simulink model "bh_CONTROL_4dof_manip_swing_balance"  (R2017a)
settings: Solver=ode4  StartTime=0.0  StopTime=44  FixedStep=0.001  RelTol=1e-5
values from neighbouring files (symbols this model uses):
  b3_damp = res_T.b3_damp    [bh_pend_solve_ODE_sys.m]
  g = res_T.g    [bh_pend_solve_ODE_sys.m]    (also in bh_pend_solve_ODE_sys_custom.m)
  Io3_xx = res_T.Io3_xx    [bh_pend_solve_ODE_sys.m]
  L3y = res_T.L3y    [bh_pend_solve_ODE_sys.m]    (also in bh_pend_solve_ODE_sys_custom.m)
  m = res_T.mass3    [bh_pend_solve_ODE_sys_custom.m]
  mass3 = res_T.mass3    [bh_pend_solve_ODE_sys.m]    (also in bh_pend_solve_ODE_sys_custom.m)
  N = 1 + N_steps    [bh_pend_solve_ODE_sys_custom.m]
undefined symbols (not defined in the file or in its folder): b1_damp, b2_damp, b4_damp, Hz, L1x, L1y, L1z, L2x, L2y, L2z, L3x, L3z, mass1, mass2, mass4, Rturn, theta1_0, theta1_dot_0, theta2_0, theta2_dot_0, theta3_0, theta3_dot_0, theta4_0, theta4_dot_0, X, Y, Z
libraries: simulink_extras x43, sm_lib x26, nesl_utility x24, simulink x7
(part 3 of 3)

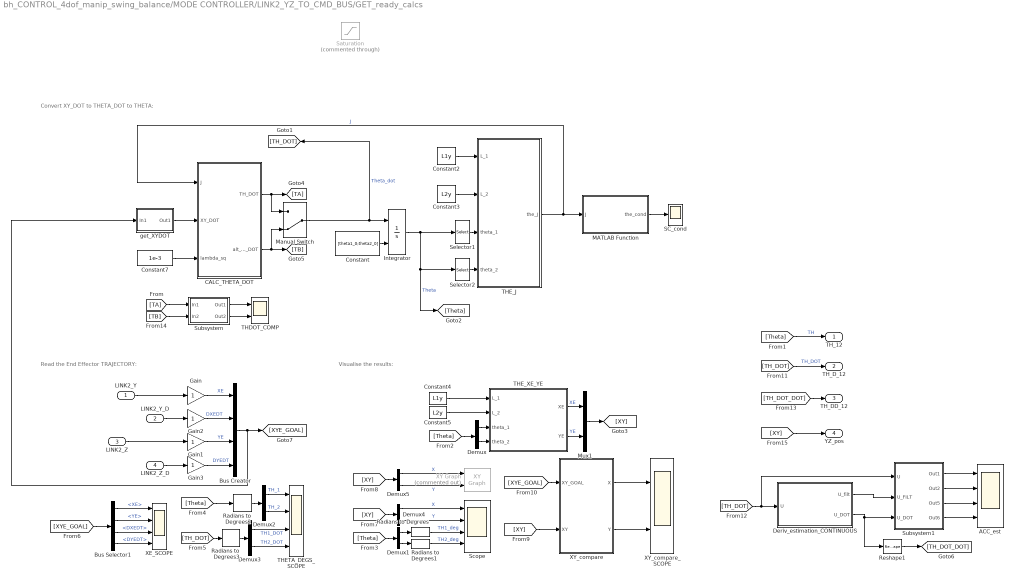
== system bh_CONTROL_4dof_manip_swing_balance/MODE CONTROLLER/LINK2_YZ_TO_CMD_BUS/GET_ready_calcs ==
  note: Visualise the results:
  note: Convert XY_DOT to THETA_DOT to THETA:
  note: Read the End Effector TRAJECTORY:
  LINK2_Y : Inport
  LINK2_Y_D : Inport  Port=2
  LINK2_Z : Inport  Port=3
  LINK2_Z_D : Inport  Port=4
  ACC_est : Scope  NumInputPorts=4
  Bus Creator : BusCreator  Inputs=4
  Bus Selector1 : BusSelector  OutputSignals=XE,YE,DXEDT,DYEDT
  CALC_THETA_DOT : MATLAB Function  TreatAsAtomicUnit=on
  Constant : Constant  Value=[theta1_0;theta2_0]  VectorParams1D=off
  Constant2 : Constant  Value=L1y
  Constant3 : Constant  Value=L2y
  Constant4 : Constant  Value=L1y
  Constant5 : Constant  Value=L2y
  Constant7 : Constant  Value=1e-3
  Demux{,1..5} (6 alike) : Demux  Outputs=2
  Deriv_estimation_CONTINUOUS : Subsystem  mask(Derivative Estimation){wn=2*pi*100, p=1, x0_val=0, v0_val=0}
      mask prompts: wn "Natural frequency, wn (rad/sec)"; p "Damping ratio, p"; x0_val "X_IC"; v0_val "X_DOT_IC"
      mask help:
      | A simple derivative estimator using a 2nd order representation between input and output.
      |
      | The integrators use a discrete FORWARd Euler rule, and a sample time needs to be specified.
      mask init:
      | str0 = sprintf('fn = %.2f [Hz]', (wn/(2*pi)));
      | str1 = sprintf('wn = %.2f', wn);
      | str2 = sprintf('p  = %.3g', p);
      | %str3 = sprintf('dt = %.2g', dt);
      | str = char(str0,str1,str2);
      mask Display: disp(str)
  Gain{,1..3} (4 alike) : Gain
  Integrator : Integrator  InitialConditionSource=external
  MATLAB Function : MATLAB Function  TreatAsAtomicUnit=on
  Manual Switch : ManualSwitch  CurrentSetting=0
  Mux1 : Mux  Inputs=2
  Radians to Degrees{,1..3} (4 alike) : simulink_extras/Transformations/Radians to Degrees
  Reshape1 : Reshape  OutputDimensionality=Column vector (2-D)
  SC_cond : Scope
  Saturation : Saturate  Commented=through  UpperLimit=6  LowerLimit=-6
  Scope : Scope  NumInputPorts=4
  Selector1 : Selector  InputPortWidth=2  IndexOptions=Index vector (dialog)  Indices=1  OutputSizes=1
  Selector2 : Selector  InputPortWidth=2  IndexOptions=Index vector (dialog)  Indices=2  OutputSizes=1
  Subsystem : Subsystem
  Subsystem1 : Subsystem
  THDOT_COMP : Scope  NumInputPorts=2
  THETA_DEGS_SCOPE : Scope  NumInputPorts=4
  THE_J : MATLAB Function  TreatAsAtomicUnit=on
  THE_XE_YE : MATLAB Function  TreatAsAtomicUnit=on
  XE_SCOPE : Scope  NumInputPorts=4
  XY Graph : simulink/Sinks/XY Graph  Commented=on  xmin=0  xmax=1.6  ymin=0  ymax=1.6  st=-1
  XY_compare : Subsystem
  XY_compare_SCOPE : Scope  NumInputPorts=2
  get_XYDOT : Subsystem
  TH_12 : Outport
  TH_D_12 : Outport  Port=2
  TH_DD_12 : Outport  Port=3
  YZ_pos : Outport  Port=4
  wires:
  XY_compare/1(X) -> XY_compare_SCOPE/1
  Constant7/1 -> CALC_THETA_DOT/3(lambda_sq)
  [XY] -> XY_compare/2(XY)
  Constant3/1 -> THE_J/2(L_2)
  Bus Selector1/2 -> XE_SCOPE/2  "<YE>"
  Subsystem/2(Out2) -> THDOT_COMP/2
  [Theta] -> Radians to Degrees2/1
  Mux1/1 -> [XY]
  Subsystem/1(Out1) -> THDOT_COMP/1
  Demux3/2 -> THETA_DEGS_SCOPE/4  "TH2_DOT"
  CALC_THETA_DOT/1(TH_DOT) -> [TA], Manual Switch/1
  [Theta] -> Demux/1
  [TB] -> Subsystem/2(In2)
  [TA] -> Subsystem/1(In1)
  Radians to Degrees1/1 -> Scope/4  "TH2_deg"
  Constant2/1 -> THE_J/1(L_1)
  CALC_THETA_DOT/2(alt_TH_DOT) -> [TB], Manual Switch/2
  XY_compare/2(Y) -> XY_compare_SCOPE/2
  THE_J/1(the_J) -> CALC_THETA_DOT/1(J), MATLAB Function/1(J)  "J"
  Radians to Degrees2/1 -> Demux2/1
  Demux5/2 -> XY Graph/2  "Y"
  [XYE_GOAL] -> XY_compare/1(XY_GOAL)
  Constant/1 -> Integrator/2
  Bus Creator/1 -> get_XYDOT/1(In1), [XYE_GOAL]
  Radians to Degrees3/1 -> Demux3/1
  Constant5/1 -> THE_XE_YE/2(L_2)
  Bus Selector1/3 -> XE_SCOPE/3  "<DXEDT>"
  Bus Selector1/4 -> XE_SCOPE/4  "<DYEDT>"
  Demux4/2 -> Scope/2  "Y"
  Demux1/1 -> Radians to Degrees/1
  Radians to Degrees/1 -> Scope/3  "TH1_deg"
  get_XYDOT/1(Out1) -> CALC_THETA_DOT/2(XY_DOT)
  Bus Selector1/1 -> XE_SCOPE/1  "<XE>"
  [XYE_GOAL] -> Bus Selector1/1
  Demux3/1 -> THETA_DEGS_SCOPE/3  "TH1_DOT"
  [TH_DOT] -> Radians to Degrees3/1
  Demux2/2 -> THETA_DEGS_SCOPE/2  "TH_2"
  [Theta] -> Demux1/1
  [XY] -> Demux5/1
  MATLAB Function/1(the_cond) -> SC_cond/1
  Demux/1 -> THE_XE_YE/3(theta_1)
  THE_XE_YE/2(YE) -> Mux1/2  "YE"
  Selector1/1 -> THE_J/3(theta_1)
  Selector2/1 -> THE_J/4(theta_2)
  Demux2/1 -> THETA_DEGS_SCOPE/1  "TH_1"
  Demux5/1 -> XY Graph/1  "X"
  Integrator/1 -> Selector2/1, [Theta], Selector1/1  "Theta"
  THE_XE_YE/1(XE) -> Mux1/1  "XE"
  [XY] -> Demux4/1
  Constant4/1 -> THE_XE_YE/1(L_1)
  Demux4/1 -> Scope/1  "X"
  Manual Switch/1 -> [TH_DOT], Integrator/1  "Theta_dot"
  Demux/2 -> THE_XE_YE/4(theta_2)
  Demux1/2 -> Radians to Degrees1/1
  [TH_DOT] -> TH_D_12/1  "TH_DOT"
  [Theta] -> TH_12/1  "TH"
  Deriv_estimation_CONTINUOUS/2(U_DOT) -> Reshape1/1, Subsystem1/3(U_DOT)
  Deriv_estimation_CONTINUOUS/1(U_filt) -> Subsystem1/2(U_FILT)
  [TH_DOT] -> Subsystem1/1(U), Deriv_estimation_CONTINUOUS/1(U)
  Reshape1/1 -> [TH_DOT_DOT]
  Subsystem1/1(Out1) -> ACC_est/1
  Subsystem1/2(Out2) -> ACC_est/2
  Subsystem1/3(Out5) -> ACC_est/3
  Subsystem1/4(Out6) -> ACC_est/4
  [TH_DOT_DOT] -> TH_DD_12/1
  Gain1/1 -> Bus Creator/3  "YE"
  Gain2/1 -> Bus Creator/2  "DXEDT"
  Gain3/1 -> Bus Creator/4  "DYEDT"
  Gain/1 -> Bus Creator/1  "XE"
  LINK2_Y/1 -> Gain/1
  LINK2_Z/1 -> Gain1/1
  LINK2_Z_D/1 -> Gain3/1
  LINK2_Y_D/1 -> Gain2/1
  [XY] -> YZ_pos/1

== system bh_CONTROL_4dof_manip_swing_balance/MODE CONTROLLER/STATE_CONTROL/BIRTH_calcs ==
  Enable : EnablePort
  Bus Creator : BusCreator  Inputs=4  OutDataTypeStr=Bus: BUS_DEF_2LINK_TRAJ
  Constant2 : Constant  Value=L1y + L2y
  Constant3 : Constant  Value=0
  Constant4 : Constant  Value=0
  Constant5 : Constant  Value=0
  LINK2_EFF_TRAJ : Outport  OutDataTypeStr=Bus: BUS_DEF_2LINK_TRAJ
  wires:
  Constant5/1 -> Bus Creator/3  "LINK2_EFF_Z_D"
  Constant2/1 -> Bus Creator/2  "LINK2_EFF_Y"
  Constant3/1 -> Bus Creator/4  "LINK2_EFF_Z"
  Constant4/1 -> Bus Creator/1  "LINK2_EFF_Y_D"
  Bus Creator/1 -> LINK2_EFF_TRAJ/1

== system bh_CONTROL_4dof_manip_swing_balance/MODE CONTROLLER/STATE_CONTROL/DO_BALANCE_calcs ==
  PMB : Inport
  Y2B : Inport  Port=2
  y_at start : Inport  Port=3
  yD_at start : Inport  Port=4
  Enable : EnablePort
  Bus Creator : BusCreator  Inputs=4  OutDataTypeStr=Bus: BUS_DEF_2LINK_TRAJ
  Constant3 : Constant  Value=0
  Constant5 : Constant  Value=0
  DO_BALANCE_sys : Subsystem  TreatAsAtomicUnit=on
  Gain1 : Gain
  Gain2 : Gain
  Scope1 : Scope
  Terminator : Terminator
  LINK2_EFF_TRAJ : Outport  OutDataTypeStr=Bus: BUS_DEF_2LINK_TRAJ
  wires:
  PMB/1 -> DO_BALANCE_sys/1(PMB)
  Y2B/1 -> DO_BALANCE_sys/2(Y2B)
  Gain1/1 -> Bus Creator/1  "LINK2_EFF_Y_D"
  Bus Creator/1 -> LINK2_EFF_TRAJ/1
  Gain2/1 -> Scope1/1, Bus Creator/2  "LINK2_EFF_Y"
  Constant5/1 -> Bus Creator/3  "LINK2_EFF_Z_D"
  Constant3/1 -> Bus Creator/4  "LINK2_EFF_Z"
  DO_BALANCE_sys/2(P) -> Gain2/1
  DO_BALANCE_sys/1(V) -> Gain1/1
  y_at start/1 -> DO_BALANCE_sys/3(y_at start)
  DO_BALANCE_sys/3(A) -> Terminator/1
  yD_at start/1 -> DO_BALANCE_sys/4(yD_at start)

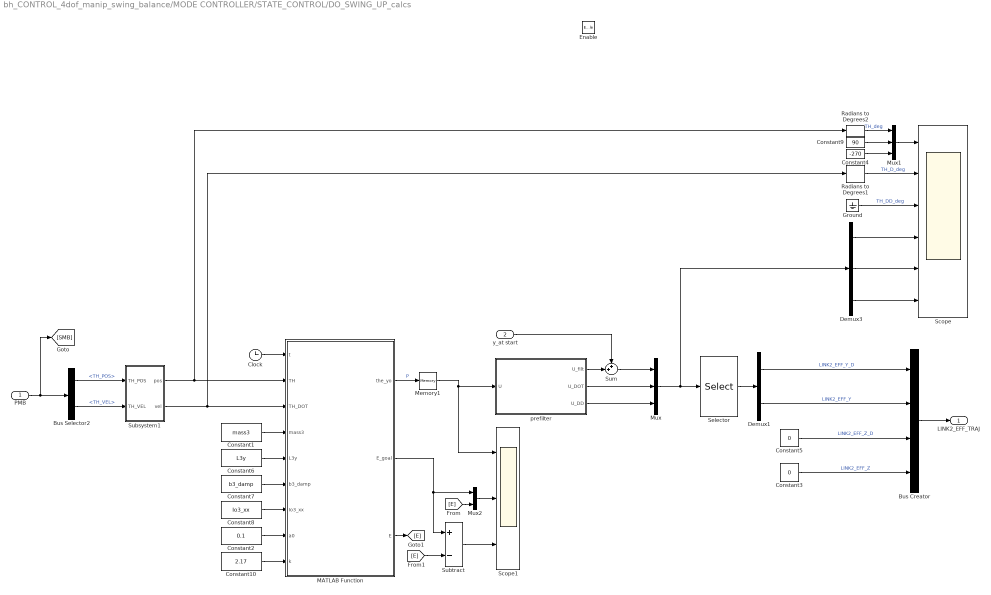
== system bh_CONTROL_4dof_manip_swing_balance/MODE CONTROLLER/STATE_CONTROL/DO_SWING_UP_calcs ==
  PMB : Inport
  y_at start : Inport  Port=2
  Enable : EnablePort
  Bus Creator : BusCreator  Inputs=4  OutDataTypeStr=Bus: BUS_DEF_2LINK_TRAJ
  Bus Selector2 : BusSelector  OutputSignals=MEAS_BUS.TH_POS,MEAS_BUS.TH_VEL
  Clock : Clock
  Constant1 : Constant  Value=mass3
  Constant10 : Constant  Value=2.17
  Constant2 : Constant  Value=0.1
  Constant3 : Constant  Value=0
  Constant4 : Constant  Value=-270
  Constant5 : Constant  Value=0
  Constant6 : Constant  Value=L3y
  Constant7 : Constant  Value=b3_damp
  Constant8 : Constant  Value=Io3_xx
  Constant9 : Constant  Value=90
  Demux1 : Demux  Outputs=2
  Demux3 : Demux  Outputs=3
  Ground : Ground
  MATLAB Function : MATLAB Function  TreatAsAtomicUnit=on
  Memory1 : Memory
  Mux : Mux  Inputs=3
  Mux1 : Mux  Inputs=3
  Mux2 : Mux  Inputs=2
  Radians to Degrees1 : simulink_extras/Transformations/Radians to Degrees
  Radians to Degrees2 : simulink_extras/Transformations/Radians to Degrees
  Scope : Scope  NumInputPorts=6
  Scope1 : Scope  NumInputPorts=3
  Selector : Selector  InputPortWidth=3  IndexOptions=Index vector (dialog)  Indices=[2 1]  OutputSizes=1
  Subsystem1 : Subsystem
  Subtract : Sum  Inputs=+-
  Sum : Sum  Inputs=++|
  prefilter : Subsystem  mask(Derivative Estimation){wn=2*pi*35, p=0.95}
      mask prompts: wn "Natural frequency, wn (rad/sec)"; p "Damping ratio, p"
      mask help:
      | A simple derivative estimator using a 2nd order representation between input and output.
      |
      | The integrators use a discrete FORWARd Euler rule, and a sample time needs to be specified.
      mask init:
      | str1 = sprintf('wn = %.2f', wn);
      | str2 = sprintf('p  = %.2f', p);
      | %str3 = sprintf('dt = %.2f', dt);
      | %str = char(str1,str2,str3);
      | %str3 = sprintf('dt = %.2f', dt);
      | str = char(str1,str2);
      mask Display: disp(str)
  LINK2_EFF_TRAJ : Outport  OutDataTypeStr=Bus: BUS_DEF_2LINK_TRAJ
  wires:
  Demux1/2 -> Bus Creator/2  "LINK2_EFF_Y"
  Demux1/1 -> Bus Creator/1  "LINK2_EFF_Y_D"
  Constant5/1 -> Bus Creator/3  "LINK2_EFF_Z_D"
  Constant3/1 -> Bus Creator/4  "LINK2_EFF_Z"
  Bus Creator/1 -> LINK2_EFF_TRAJ/1
  Clock/1 -> MATLAB Function/1(t)
  Mux1/1 -> Scope/1
  Constant10/1 -> MATLAB Function/9(k)
  Mux2/1 -> Scope1/2
  Demux3/2 -> Scope/5
  Constant6/1 -> MATLAB Function/5(L3y)
  Subtract/1 -> Scope1/3
  prefilter/1(U_filt) -> Sum/2
  prefilter/3(U_DD) -> Mux/3
  Constant8/1 -> MATLAB Function/7(Io3_xx)
  Ground/1 -> Scope/3  "TH_DD_deg"
  MATLAB Function/2(E_goal) -> Mux2/1, Subtract/1
  Demux3/3 -> Scope/6
  Constant7/1 -> MATLAB Function/6(b3_damp)
  Constant1/1 -> MATLAB Function/4(mass3)
  Constant2/1 -> MATLAB Function/8(a0)
  Constant9/1 -> Mux1/2
  Demux3/1 -> Scope/4
  Radians to Degrees2/1 -> Mux1/1  "TH_deg"
  MATLAB Function/1(the_yo) -> Memory1/1  "P"
  Radians to Degrees1/1 -> Scope/2  "TH_D_deg"
  prefilter/2(U_DOT) -> Mux/2
  PMB/1 -> [SMB], Bus Selector2/1
  Mux/1 -> Selector/1, Demux3/1
  Bus Selector2/1 -> Subsystem1/1(TH_POS)  "<TH_POS>"
  Bus Selector2/2 -> Subsystem1/2(TH_VEL)  "<TH_VEL>"
  Subsystem1/1(pos) -> MATLAB Function/2(TH), Radians to Degrees2/1
  Subsystem1/2(vel) -> MATLAB Function/3(TH_DOT), Radians to Degrees1/1
  Sum/1 -> Mux/1
  y_at start/1 -> Sum/1
  Selector/1 -> Demux1/1
  Constant4/1 -> Mux1/3
  Memory1/1 -> prefilter/1(U), Scope1/1
  MATLAB Function/3(E) -> [E]
  [E] -> Subtract/2
  [E] -> Mux2/2

== system bh_CONTROL_4dof_manip_swing_balance/MODE CONTROLLER/STATE_CONTROL/DO_moving_to_ready_calcs ==
  Enable : EnablePort
  BIRTH_moves_to_READY1 : Subsystem
  LINK2_traj : Outport  OutDataTypeStr=Bus: BUS_DEF_2LINK_TRAJ
  wires:
  BIRTH_moves_to_READY1/1(LINK2_EFF_TRAJ) -> LINK2_traj/1

== system bh_CONTROL_4dof_manip_swing_balance/MODE CONTROLLER/STATE_CONTROL/Subsystem ==
  PMB : Inport
  Bus Creator : BusCreator  Inputs=2
  Bus Selector : BusSelector  OutputSignals=MEAS_BUS.TH_POS
  Demux : Demux  Outputs=2
  Deriv_estimation_CONTINUOUS : Subsystem  mask(Derivative Estimation){wn=2*pi*100, p=1, x0_val=0, v0_val=0}
      mask prompts: wn "Natural frequency, wn (rad/sec)"; p "Damping ratio, p"; x0_val "X_IC"; v0_val "X_DOT_IC"
      mask help:
      | A simple derivative estimator using a 2nd order representation between input and output.
      |
      | The integrators use a discrete FORWARd Euler rule, and a sample time needs to be specified.
      mask init:
      | str0 = sprintf('fn = %.2f [Hz]', (wn/(2*pi)));
      | str1 = sprintf('wn = %.2f', wn);
      | str2 = sprintf('p  = %.3g', p);
      | %str3 = sprintf('dt = %.2g', dt);
      | str = char(str0,str1,str2);
      mask Display: disp(str)
  LINK2_EFF_YZ_from_THETA : Subsystem
  Selector1 : Selector  InputPortWidth=4  IndexOptions=Index vector (dialog)  Indices=[1,2]  OutputSizes=1
  Terminator : Terminator
  Terminator1 : Terminator
  Y2 : Outport
  Y2_D : Outport  Port=2
  Y2_Bus : Outport  Port=3
  wires:
  PMB/1 -> Bus Selector/1
  Bus Selector/1 -> Selector1/1  "<TH_POS>"
  Selector1/1 -> Demux/1
  Demux/1 -> LINK2_EFF_YZ_from_THETA/1(TH1)
  Demux/2 -> LINK2_EFF_YZ_from_THETA/2(TH2)
  LINK2_EFF_YZ_from_THETA/2(Z2_EFF) -> Terminator/1
  LINK2_EFF_YZ_from_THETA/1(Y2_EFF) -> Deriv_estimation_CONTINUOUS/1(U), Bus Creator/1, Y2/1  "Y2"
  Deriv_estimation_CONTINUOUS/1(U_filt) -> Terminator1/1
  Bus Creator/1 -> Y2_Bus/1
  Deriv_estimation_CONTINUOUS/2(U_DOT) -> Y2_D/1, Bus Creator/2  "Y2_D"

== system bh_CONTROL_4dof_manip_swing_balance/MODE CONTROLLER/STATE_CONTROL/Subsystem1 ==
  TH_POS : Inport
  TH_VEL : Inport  Port=2
  Mux : Mux  Inputs=2
  Selector1 : Selector  InputPortWidth=4  IndexOptions=Index vector (dialog)  Indices=[1 2 3]  OutputSizes=1
  Selector2 : Selector  InputPortWidth=4  IndexOptions=Index vector (dialog)  Indices=[1 2 3]  OutputSizes=1
  Sum of Elements : Sum  Inputs=+
  Sum of Elements1 : Sum  Inputs=+
  pos : Outport
  vel : Outport  Port=2
  PV : Outport  Port=3
  wires:
  TH_POS/1 -> Selector2/1
  Sum of Elements/1 -> Mux/1, pos/1
  Selector2/1 -> Sum of Elements/1
  TH_VEL/1 -> Selector1/1
  Selector1/1 -> Sum of Elements1/1
  Sum of Elements1/1 -> Mux/2, vel/1
  Mux/1 -> PV/1

== system bh_CONTROL_4dof_manip_swing_balance/SIMULINK_MODEL/inside_MCKGQ/Subsystem ==
  iTH1 : Inport
  iTH2 : Inport  Port=2
  iTH3 : Inport  Port=3
  iTH4 : Inport  Port=4
  iTH1D : Inport  Port=5
  iTH2D : Inport  Port=6
  iTH3D : Inport  Port=7
  iTH4D : Inport  Port=8
  Bus Creator : BusCreator  Inputs=10
  Bus Selector : BusSelector  OutputSignals=TH1,TH2,TH3,TH4,TH1D,TH2D,TH3D,TH4D
  Mux : Mux
  Mux1 : Mux
  Reshape : Reshape  OutputDimensionality=Column vector (2-D)
  Reshape1 : Reshape  OutputDimensionality=Column vector (2-D)
  Terminator : Terminator
  TH1 : Outport
  TH2 : Outport  Port=2
  TH3 : Outport  Port=3
  TH1D : Outport  Port=4
  TH2D : Outport  Port=5
  TH3D : Outport  Port=6
  TH4D : Outport  Port=7
  TH_BUS : Outport  Port=8
  wires:
  iTH2/1 -> Bus Creator/3, Mux/2  "TH2"
  iTH1/1 -> Bus Creator/2, Mux/1  "TH1"
  iTH2D/1 -> Bus Creator/7, Mux1/2  "TH2D"
  iTH1D/1 -> Bus Creator/6, Mux1/1  "TH1D"
  Mux/1 -> Reshape/1
  Mux1/1 -> Reshape1/1
  Reshape/1 -> Bus Creator/1  "theta_col"
  Reshape1/1 -> Bus Creator/10  "theta_DOT_col"
  Bus Creator/1 -> TH_BUS/1, Bus Selector/1
  iTH3D/1 -> Bus Creator/8, Mux1/3  "TH3D"
  iTH3/1 -> Bus Creator/4, Mux/3  "TH3"
  Bus Selector/1 -> TH1/1  "<TH1>"
  Bus Selector/2 -> TH2/1  "<TH2>"
  Bus Selector/3 -> TH3/1  "<TH3>"
  Bus Selector/5 -> TH1D/1  "<TH1D>"
  Bus Selector/6 -> TH2D/1  "<TH2D>"
  Bus Selector/7 -> TH3D/1  "<TH3D>"
  iTH4/1 -> Bus Creator/5, Mux/4  "TH4"
  iTH4D/1 -> Bus Creator/9, Mux1/4  "TH4D"
  Bus Selector/4 -> Terminator/1  "<TH4>"
  Bus Selector/8 -> TH4D/1  "<TH4D>"

== system bh_CONTROL_4dof_manip_swing_balance/SIMULINK_MODEL/inside_MCKGQ/Subsystem1 ==
  M : Inport
  C : Inport  Port=2
  K : Inport  Port=3
  G : Inport  Port=4
  Q : Inport  Port=5
  T : Inport  Port=6
  Bus Selector : BusSelector  OutputSignals=theta_DOT_col
  Bus Selector1 : BusSelector  OutputSignals=theta_col
  Demux : Demux
  MATLAB Function : MATLAB Function  TreatAsAtomicUnit=on
  Product : Product  Multiplication=Matrix(*)
  Product1 : Product  Multiplication=Matrix(*)
  Product2 : Product  Inputs=/  Multiplication=Matrix(*)
  Product3 : Product  Multiplication=Matrix(*)
  SC_cond : Scope
  Sum : Sum  Inputs=+|+|+
  Sum1 : Sum  Inputs=|-+
  TH1_DD : Outport
  TH2_DD : Outport  Port=2
  TH3_DD : Outport  Port=3
  TH4_DD : Outport  Port=4
  wires:
  T/1 -> [T]
  C/1 -> Product/1
  [T] -> Bus Selector/1
  Bus Selector/1 -> Product/2  "<theta_DOT_col>"
  K/1 -> Product1/1
  [T] -> Bus Selector1/1
  Bus Selector1/1 -> Product1/2  "<theta_col>"
  Q/1 -> Sum1/2
  Product1/1 -> Sum/2
  G/1 -> Sum/3
  Product/1 -> Sum/1
  Sum/1 -> Sum1/1
  M/1 -> [M], Product2/1
  Product2/1 -> Product3/1
  Sum1/1 -> Product3/2
  Product3/1 -> Demux/1
  Demux/1 -> TH1_DD/1
  Demux/2 -> TH2_DD/1
  MATLAB Function/1(the_cond) -> SC_cond/1
  Demux/3 -> TH3_DD/1
  Demux/4 -> TH4_DD/1
  [M] -> MATLAB Function/1(M)

== system bh_CONTROL_4dof_manip_swing_balance/MODE CONTROLLER/LINK2_YZ_TO_CMD_BUS/GET_ready_calcs/Deriv_estimation_CONTINUOUS ==
  note: Y = U *     wn^2/( s^2 + 2*p*wn*s + wn^2)
      | Y*( s^2 + 2*p*wn*s + wn^2) = U * wn^2
      |
      | y'' + y'*2*p*wn + y*wn^2 = U*wn^2
  U : Inport
  Constant : Constant  Value=x0_val
  Constant1 : Constant  Value=v0_val
  Gain : Gain  Gain=2*p*wn
  Gain1 : Gain  Gain=wn^2
  Gain2 : Gain  Gain=wn^2
  Integrator : Integrator  InitialConditionSource=external
  Integrator1 : Integrator  InitialConditionSource=external
  Sum : Sum  Inputs=|+--
  U_filt : Outport
  U_DOT : Outport  Port=2
  wires:
  Integrator/1 -> Integrator1/1, [Y_DOT], Gain/1  "y_dot"
  Sum/1 -> Integrator/1  "y_dot_dot"
  Integrator1/1 -> U_filt/1, Gain1/1  "y"
  U/1 -> Gain2/1
  Gain2/1 -> Sum/1
  Gain/1 -> Sum/3
  Gain1/1 -> Sum/2
  [Y_DOT] -> U_DOT/1
  Constant/1 -> Integrator1/2
  Constant1/1 -> Integrator/2

== system bh_CONTROL_4dof_manip_swing_balance/MODE CONTROLLER/LINK2_YZ_TO_CMD_BUS/GET_ready_calcs/Subsystem ==
  In1 : Inport
  In2 : Inport  Port=2
  Mux2 : Mux  Inputs=2
  Reshape : Reshape  OutputDimensionality=Column vector (2-D)
  Reshape1 : Reshape  OutputDimensionality=Column vector (2-D)
  Selector : Selector  InputPortWidth=4  IndexOptions=Index vector (dialog)  Indices=[1 3]  OutputSizes=1
  Selector1 : Selector  InputPortWidth=4  IndexOptions=Index vector (dialog)  Indices=[2 4]  OutputSizes=1
  Out1 : Outport
  Out2 : Outport  Port=2
  wires:
  In1/1 -> Reshape/1
  In2/1 -> Reshape1/1
  Reshape/1 -> Mux2/1
  Reshape1/1 -> Mux2/2
  Selector1/1 -> Out2/1
  Selector/1 -> Out1/1
  Mux2/1 -> Selector/1, Selector1/1

== system bh_CONTROL_4dof_manip_swing_balance/MODE CONTROLLER/LINK2_YZ_TO_CMD_BUS/GET_ready_calcs/Subsystem1 ==
  U : Inport
  U_FILT : Inport  Port=2
  U_DOT : Inport  Port=3
  Demux : Demux  Outputs=2
  Mux2 : Mux  Inputs=2
  Reshape : Reshape  OutputDimensionality=Column vector (2-D)
  Reshape2 : Reshape  OutputDimensionality=Column vector (2-D)
  Selector : Selector  InputPortWidth=4  IndexOptions=Index vector (dialog)  Indices=[1 3]  OutputSizes=1
  Selector1 : Selector  InputPortWidth=4  IndexOptions=Index vector (dialog)  Indices=[2 4]  OutputSizes=1
  Out1 : Outport
  Out2 : Outport  Port=2
  Out5 : Outport  Port=3
  Out6 : Outport  Port=4
  wires:
  U_FILT/1 -> Reshape/1
  U_DOT/1 -> Demux/1
  Selector1/1 -> Out2/1
  Selector/1 -> Out1/1
  Mux2/1 -> Selector1/1, Selector/1
  U/1 -> Reshape2/1
  Reshape/1 -> Mux2/2
  Reshape2/1 -> Mux2/1
  Demux/1 -> Out5/1
  Demux/2 -> Out6/1

== system bh_CONTROL_4dof_manip_swing_balance/MODE CONTROLLER/LINK2_YZ_TO_CMD_BUS/GET_ready_calcs/XY_compare ==
  XY_GOAL : Inport
  XY : Inport  Port=2
  Bus Selector1 : BusSelector  OutputSignals=XE,YE
  Demux : Demux  Outputs=2
  Mux : Mux  Inputs=2
  Mux1 : Mux  Inputs=2
  X : Outport
  Y : Outport  Port=2
  wires:
  XY_GOAL/1 -> Bus Selector1/1
  XY/1 -> Demux/1
  Bus Selector1/1 -> Mux/1  "<XE>"
  Demux/1 -> Mux/2
  Bus Selector1/2 -> Mux1/1  "<YE>"
  Demux/2 -> Mux1/2
  Mux/1 -> X/1
  Mux1/1 -> Y/1

== system bh_CONTROL_4dof_manip_swing_balance/MODE CONTROLLER/LINK2_YZ_TO_CMD_BUS/GET_ready_calcs/get_XYDOT ==
  In1 : Inport
  Bus Selector2 : BusSelector  OutputSignals=DXEDT,DYEDT
  Mux2 : Mux  Inputs=2
  Reshape : Reshape  OutputDimensionality=Column vector (2-D)
  Out1 : Outport
  wires:
  Bus Selector2/1 -> Mux2/1  "<DXEDT>"
  Bus Selector2/2 -> Mux2/2  "<DYEDT>"
  In1/1 -> Bus Selector2/1
  Mux2/1 -> Reshape/1
  Reshape/1 -> Out1/1  "XY_DOT"

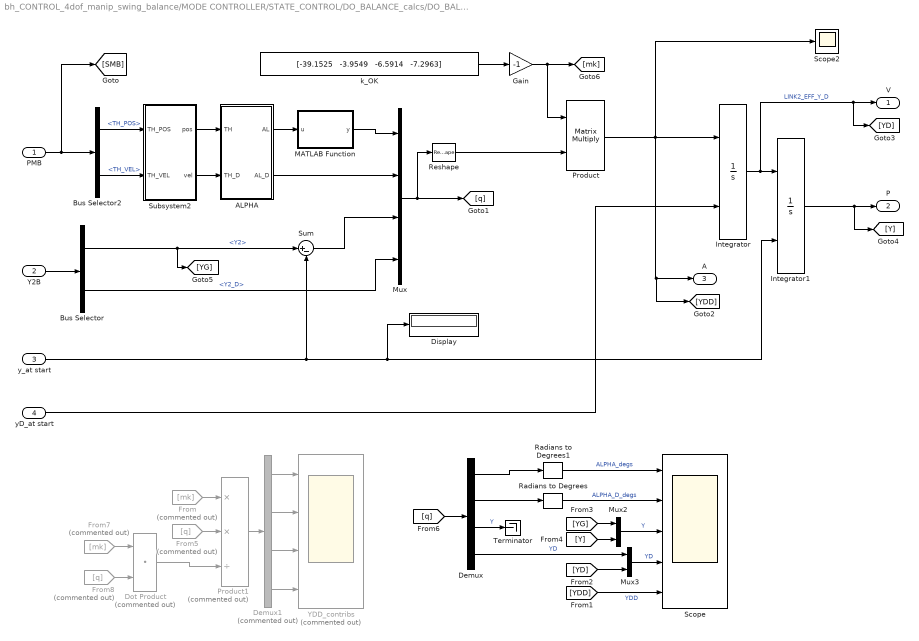
== system bh_CONTROL_4dof_manip_swing_balance/MODE CONTROLLER/STATE_CONTROL/DO_BALANCE_calcs/DO_BALANCE_sys ==
  PMB : Inport
  Y2B : Inport  Port=2
  y_at start : Inport  Port=3
  yD_at start : Inport  Port=4
  ALPHA : Subsystem
  Bus Selector : BusSelector  OutputSignals=Y2,Y2_D
  Bus Selector2 : BusSelector  OutputSignals=MEAS_BUS.TH_POS,MEAS_BUS.TH_VEL
  Demux : Demux
  Demux1 : Demux  Commented=on
  Display : Display
  Dot Product : DotProduct  Commented=on  InputSameDT=on  OutDataTypeStr=Inherit: Inherit via internal rule
  From : From  Commented=on  GotoTag=mk
  From5 : From  Commented=on  GotoTag=q
  From7 : From  Commented=on  GotoTag=mk
  From8 : From  Commented=on  GotoTag=q
  Gain : Gain  Gain=-1
  Integrator : Integrator  InitialConditionSource=external
  Integrator1 : Integrator  InitialConditionSource=external
  MATLAB Function : MATLAB Function  TreatAsAtomicUnit=on
  Mux : Mux
  Mux2 : Mux  Inputs=2
  Mux3 : Mux  Inputs=2
  Product : Product  Multiplication=Matrix(*)
  Product1 : Product  Commented=on  Inputs=**/
  Radians to Degrees : simulink_extras/Transformations/Radians to Degrees
  Radians to Degrees1 : simulink_extras/Transformations/Radians to Degrees
  Reshape : Reshape  OutputDimensionality=Column vector (2-D)
  Scope : Scope  NumInputPorts=5
  Scope2 : Scope
  Subsystem2 : Subsystem
  Sum : Sum  Inputs=|+-
  Terminator : Terminator
  YDD_contribs : Scope  Commented=on  NumInputPorts=4
  k_OK : Constant  Value="[-39.1525   -3.9549   -6.5914   -7.2963]"  VectorParams1D=off
  V : Outport
  P : Outport  Port=2
  A : Outport  Port=3
  wires:
  Subsystem2/1(pos) -> ALPHA/1(TH)
  Bus Selector2/2 -> Subsystem2/2(TH_VEL)  "<TH_VEL>"
  PMB/1 -> [SMB], Bus Selector2/1
  Bus Selector2/1 -> Subsystem2/1(TH_POS)  "<TH_POS>"
  Mux/1 -> Reshape/1, [q]
  Reshape/1 -> Product/2
  Product/1 -> Integrator/1, [YDD], A/1, Scope2/1
  y_at start/1 -> Integrator1/2, Display/1, Sum/2
  Radians to Degrees1/1 -> Scope/1  "ALPHA_degs"
  Radians to Degrees/1 -> Scope/2  "ALPHA_D_degs"
  MATLAB Function/1(y) -> Mux/1
  ALPHA/1(AL) -> MATLAB Function/1(u)
  Subsystem2/2(vel) -> ALPHA/2(TH_D)
  Y2B/1 -> Bus Selector/1
  Bus Selector/1 -> [YG], Sum/1  "<Y2>"
  Integrator/1 -> [YD], V/1, Integrator1/1  "LINK2_EFF_Y_D"
  Demux/4 -> Mux3/1  "YD"
  Demux/3 -> Terminator/1  "Y"
  Demux/2 -> Radians to Degrees/1
  Demux/1 -> Radians to Degrees1/1
  [q] -> Demux/1
  Sum/1 -> Mux/3
  Integrator1/1 -> [Y], P/1
  [YDD] -> Scope/5  "YDD"
  Mux3/1 -> Scope/4  "YD"
  Mux2/1 -> Scope/3  "Y"
  [YD] -> Mux3/2
  [YG] -> Mux2/1
  [Y] -> Mux2/2
  Gain/1 -> [mk], Product/1
  From5/1 -> Product1/2
  From/1 -> Product1/1
  Product1/1 -> Demux1/1
  Demux1/4 -> YDD_contribs/4
  Demux1/3 -> YDD_contribs/3
  Demux1/2 -> YDD_contribs/2
  Demux1/1 -> YDD_contribs/1
  From8/1 -> Dot Product/2
  From7/1 -> Dot Product/1
  Dot Product/1 -> Product1/3
  ALPHA/2(AL_D) -> Mux/2
  Bus Selector/2 -> Mux/4  "<Y2_D>"
  k_OK/1 -> Gain/1
  yD_at start/1 -> Integrator/2

== system bh_CONTROL_4dof_manip_swing_balance/MODE CONTROLLER/STATE_CONTROL/DO_SWING_UP_calcs/Subsystem1 ==
  TH_POS : Inport
  TH_VEL : Inport  Port=2
  Selector1 : Selector  InputPortWidth=4  IndexOptions=Index vector (dialog)  Indices=[1 2 3]  OutputSizes=1
  Selector2 : Selector  InputPortWidth=4  IndexOptions=Index vector (dialog)  Indices=[1 2 3]  OutputSizes=1
  Sum of Elements : Sum  Inputs=+
  Sum of Elements1 : Sum  Inputs=+
  pos : Outport
  vel : Outport  Port=2
  wires:
  TH_POS/1 -> Selector2/1
  Sum of Elements/1 -> pos/1
  Selector2/1 -> Sum of Elements/1
  TH_VEL/1 -> Selector1/1
  Selector1/1 -> Sum of Elements1/1
  Sum of Elements1/1 -> vel/1

== system bh_CONTROL_4dof_manip_swing_balance/MODE CONTROLLER/STATE_CONTROL/DO_SWING_UP_calcs/prefilter ==
  note: Y = U *     wn^2/( s^2 + 2*p*wn*s + wn^2)
      | Y*( s^2 + 2*p*wn*s + wn^2) = U * wn^2
      |
      | y'' + y'*2*p*wn + y*wn^2 = U*wn^2
  U : Inport
  Gain : Gain  Gain=2*p*wn
  Gain1 : Gain  Gain=wn^2
  Gain2 : Gain  Gain=wn^2
  Integrator : Integrator
  Integrator1 : Integrator
  Sum : Sum  Inputs=|+--
  U_filt : Outport
  U_DOT : Outport  Port=2
  U_DD : Outport  Port=3
  wires:
  Integrator/1 -> Integrator1/1, [Y_DOT], Gain/1  "y_dot"
  Sum/1 -> [Y_DD], Integrator/1  "y_dot_dot"
  Integrator1/1 -> Gain1/1, U_filt/1  "y"
  U/1 -> Gain2/1
  Gain2/1 -> Sum/1
  Gain/1 -> Sum/3
  Gain1/1 -> Sum/2
  [Y_DOT] -> U_DOT/1
  [Y_DD] -> U_DD/1

== system bh_CONTROL_4dof_manip_swing_balance/MODE CONTROLLER/STATE_CONTROL/DO_moving_to_ready_calcs/BIRTH_moves_to_READY1 ==
  Bus Creator : BusCreator  Inputs=4  OutDataTypeStr=Bus: BUS_DEF_2LINK_TRAJ
  Constant : Constant  Value=L1y + L2y
  Constant1 : Constant  Value=0
  Constant2 : Constant  Value=-0.05
  Constant3 : Constant  Value=0
  X : Integrator  InitialConditionSource=external
  Y : Integrator  InitialConditionSource=external
  LINK2_EFF_TRAJ : Outport
  wires:
  Bus Creator/1 -> LINK2_EFF_TRAJ/1
  Constant/1 -> X/2
  Constant1/1 -> Y/2
  Constant2/1 -> Bus Creator/1, X/1  "LINK2_EFF_Y_D"
  Constant3/1 -> Bus Creator/3, Y/1  "LINK2_EFF_Z_D"
  X/1 -> Bus Creator/2  "LINK2_EFF_Y"
  Y/1 -> Bus Creator/4  "LINK2_EFF_Z"

== system bh_CONTROL_4dof_manip_swing_balance/MODE CONTROLLER/STATE_CONTROL/Subsystem/Deriv_estimation_CONTINUOUS ==
  note: Y = U *     wn^2/( s^2 + 2*p*wn*s + wn^2)
      | Y*( s^2 + 2*p*wn*s + wn^2) = U * wn^2
      |
      | y'' + y'*2*p*wn + y*wn^2 = U*wn^2
  U : Inport
  Constant : Constant  Value=x0_val
  Constant1 : Constant  Value=v0_val
  Gain : Gain  Gain=2*p*wn
  Gain1 : Gain  Gain=wn^2
  Gain2 : Gain  Gain=wn^2
  Integrator : Integrator  InitialConditionSource=external
  Integrator1 : Integrator  InitialConditionSource=external
  Sum : Sum  Inputs=|+--
  U_filt : Outport
  U_DOT : Outport  Port=2
  wires:
  Integrator/1 -> Integrator1/1, [Y_DOT], Gain/1  "y_dot"
  Sum/1 -> Integrator/1  "y_dot_dot"
  Integrator1/1 -> U_filt/1, Gain1/1  "y"
  U/1 -> Gain2/1
  Gain2/1 -> Sum/1
  Gain/1 -> Sum/3
  Gain1/1 -> Sum/2
  [Y_DOT] -> U_DOT/1
  Constant/1 -> Integrator1/2
  Constant1/1 -> Integrator/2

== system bh_CONTROL_4dof_manip_swing_balance/MODE CONTROLLER/STATE_CONTROL/Subsystem/LINK2_EFF_YZ_from_THETA ==
  TH1 : Inport
  TH2 : Inport  Port=2
  Constant4 : Constant  Value=L1y
  Constant5 : Constant  Value=L2y
  THE_XE_YE : MATLAB Function  TreatAsAtomicUnit=on
  Y2_EFF : Outport
  Z2_EFF : Outport  Port=2
  wires:
  Constant5/1 -> THE_XE_YE/2(L_2)
  THE_XE_YE/2(YE) -> Z2_EFF/1  "Z2_EFF"
  TH2/1 -> THE_XE_YE/4(theta_2)
  Constant4/1 -> THE_XE_YE/1(L_1)
  THE_XE_YE/1(XE) -> Y2_EFF/1  "Y2_EFF"
  TH1/1 -> THE_XE_YE/3(theta_1)

== system bh_CONTROL_4dof_manip_swing_balance/MODE CONTROLLER/STATE_CONTROL/DO_BALANCE_calcs/DO_BALANCE_sys/ALPHA ==
  TH : Inport
  TH_D : Inport  Port=2
  Constant : Constant  Value=pi/2
  Gain : Gain  Gain=-1
  Sum : Sum  Inputs=+-|
  AL : Outport
  AL_D : Outport  Port=2
  wires:
  TH/1 -> Sum/2
  Constant/1 -> Sum/1
  Sum/1 -> AL/1
  TH_D/1 -> Gain/1
  Gain/1 -> AL_D/1

== system bh_CONTROL_4dof_manip_swing_balance/MODE CONTROLLER/STATE_CONTROL/DO_BALANCE_calcs/DO_BALANCE_sys/Subsystem2 ==
  TH_POS : Inport
  TH_VEL : Inport  Port=2
  Selector1 : Selector  InputPortWidth=4  IndexOptions=Index vector (dialog)  Indices=[1 2 3]  OutputSizes=1
  Selector2 : Selector  InputPortWidth=4  IndexOptions=Index vector (dialog)  Indices=[1 2 3]  OutputSizes=1
  Sum of Elements : Sum  Inputs=+
  Sum of Elements1 : Sum  Inputs=+
  pos : Outport
  vel : Outport  Port=2
  wires:
  TH_POS/1 -> Selector2/1
  Sum of Elements/1 -> pos/1
  Selector2/1 -> Sum of Elements/1
  TH_VEL/1 -> Selector1/1
  Selector1/1 -> Sum of Elements1/1
  Sum of Elements1/1 -> vel/1

== matlab function bh_CONTROL_4dof_manip_swing_balance/SIMULINK_MODEL/inside_MCKGQ/MCKGQ ==
  data: L1X_s input; M output; L2X_s input; L3X_s input; L1Y_s input; L2Y_s input; L3Y_s input; L1Z_s input; L2Z_s input; L3Z_s input; R4_s input; TH1_s input; TH2_s input; TH3_s input; TH1_s_D input; TH2_s_D input; TH3_s_D input; TH4_s_D input; b1_s input; b2_s input; b3_s input; b4_s input; g_s input; m1_s input; m2_s input; m3_s input; m4_s input; taum1_s input; taum2_s input; taum3_s input; taum4_s input; C output; K output; G output; Q output
function [M,C,K,G,Q] = MCKGQ(L1X_s,L2X_s,L3X_s,L1Y_s,L2Y_s,L3Y_s,L1Z_s,L2Z_s,L3Z_s,R4_s,TH1_s,TH2_s,TH3_s,TH1_s_D,TH2_s_D,TH3_s_D,TH4_s_D,b1_s,b2_s,b3_s,b4_s,g_s,m1_s,m2_s,m3_s,m4_s,taum1_s,taum2_s,taum3_s,taum4_s)
%#codegen

%    This function was generated by the Symbolic Math Toolbox version 7.2.
%    27-Mar-2017 09:25:14

M = reshape([L1Y_s.^2.*m1_s.*(1.0./3.0)+L1Y_s.^2.*m2_s+L1Y_s.^2.*m3_s+L2Y_s.^2.*m2_s.*(1.0./3.0)+L2Y_s.^2.*m3_s+L3Y_s.^2.*m3_s.*(1.0./3.0)+L1Z_s.^2.*m1_s.*(1.0./1.2e1)+L2Z_s.^2.*m2_s.*(1.0./1.2e1)+L3Z_s.^2.*m3_s.*(1.0./1.2e1)+L1Y_s.*L2Y_s.*m2_s.*cos(TH2_s)+L1Y_s.*L2Y_s.*m3_s.*cos(TH2_s).*2.0+L2Y_s.*L3Y_s.*m3_s.*cos(TH3_s)+L1Y_s.*L3Y_s.*m3_s.*cos(TH2_s+TH3_s),L2Y_s.^2.*m2_s.*(1.0./3.0)+L2Y_s.^2.*m3_s+L3Y_s.^2.*m3_s.*(1.0./3.0)+L2Z_s.^2.*m2_s.*(1.0./1.2e1)+L3Z_s.^2.*m3_s.*(1.0./1.2e1)+L1Y_s.*L2Y_s.*m2_s.*cos(TH2_s).*(1.0./2.0)+L1Y_s.*L2Y_s.*m3_s.*cos(TH2_s)+L2Y_s.*L3Y_s.*m3_s.*cos(TH3_s)+L1Y_s.*L3Y_s.*m3_s.*cos(TH2_s+TH3_s).*(1.0./2.0),m3_s.*(L3Y_s.^2.*4.0+L3Z_s.^2+L1Y_s.*L3Y_s.*cos(TH2_s+TH3_s).*6.0+L2Y_s.*L3Y_s.*cos(TH3_s).*6.0).*(1.0./1.2e1),0.0,L2Y_s.^2.*m2_s.*(1.0./3.0)+L2Y_s.^2.*m3_s+L3Y_s.^2.*m3_s.*(1.0./3.0)+L2Z_s.^2.*m2_s.*(1.0./1.2e1)+L3Z_s.^2.*m3_s.*(1.0./1.2e1)+L1Y_s.*L2Y_s.*m2_s.*cos(TH2_s).*(1.0./2.0)+L1Y_s.*L2Y_s.*m3_s.*cos(TH2_s)+L2Y_s.*L3Y_s.*m3_s.*cos(TH3_s)+L1Y_s.*L3Y_s.*m3_s.*cos(TH2_s+TH3_s).*(1.0./2.0),L2Y_s.^2.*m2_s.*(1.0./3.0)+L2Y_s.^2.*m3_s+L3Y_s.^2.*m3_s.*(1.0./3.0)+L2Z_s.^2.*m2_s.*(1.0./1.2e1)+L3Z_s.^2.*m3_s.*(1.0./1.2e1)+L2Y_s.*L3Y_s.*m3_s.*cos(TH3_s),m3_s.*(L3Y_s.^2.*4.0+L3Z_s.^2+L2Y_s.*L3Y_s.*cos(TH3_s).*6.0).*(1.0./1.2e1),0.0,m3_s.*(L3Y_s.^2.*4.0+L3Z_s.^2+L1Y_s.*L3Y_s.*cos(TH2_s+TH3_s).*6.0+L2Y_s.*L3Y_s.*cos(TH3_s).*6.0).*(1.0./1.2e1),m3_s.*(L3Y_s.^2.*4.0+L3Z_s.^2+L2Y_s.*L3Y_s.*cos(TH3_s).*6.0).*(1.0./1.2e1),m3_s.*(L3Y_s.^2.*4.0+L3Z_s.^2).*(1.0./1.2e1),0.0,0.0,0.0,0.0,L1X_s.^2.*m1_s.*(1.0./1.2e1)+L2X_s.^2.*m2_s.*(1.0./1.2e1)+L3X_s.^2.*m3_s.*(1.0./1.2e1)+L1Y_s.^2.*m1_s.*(1.0./6.0)+L1Y_s.^2.*m2_s.*(1.0./2.0)+L1Y_s.^2.*m3_s.*(1.0./2.0)+L2Y_s.^2.*m2_s.*(1.0./6.0)+L2Y_s.^2.*m3_s.*(1.0./2.0)+L3Y_s.^2.*m3_s.*(1.0./6.0)+L1Z_s.^2.*m1_s.*(1.0./2.4e1)+L2Z_s.^2.*m2_s.*(1.0./2.4e1)+L3Z_s.^2.*m3_s.*(1.0./2.4e1)+R4_s.^2.*m4_s.*(1.0./2.0)+L3Y_s.^2.*m3_s.*cos(TH1_s.*2.0+TH2_s.*2.0+TH3_s.*2.0).*(1.0./6.0)-L3Z_s.^2.*m3_s.*cos(TH1_s.*2.0+TH2_s.*2.0+TH3_s.*2.0).*(1.0./2.4e1)+L1Y_s.^2.*m1_s.*cos(TH1_s.*2.0).*(1.0./6.0)+L1Y_s.^2.*m2_s.*cos(TH1_s.*2.0).*(1.0./2.0)+L1Y_s.^2.*m3_s.*cos(TH1_s.*2.0).*(1.0./2.0)-L1Z_s.^2.*m1_s.*cos(TH1_s.*2.0).*(1.0./2.4e1)+L2Y_s.^2.*m2_s.*cos(TH1_s.*2.0+TH2_s.*2.0).*(1.0./6.0)+L2Y_s.^2.*m3_s.*cos(TH1_s.*2.0+TH2_s.*2.0).*(1.0./2.0)-L2Z_s.^2.*m2_s.*cos(TH1_s.*2.0+TH2_s.*2.0).*(1.0./2.4e1)+L1Y_s.*L2Y_s.*m2_s.*cos(TH2_s).*(1.0./2.0)+L1Y_s.*L2Y_s.*m3_s.*cos(TH2_s)+L2Y_s.*L3Y_s.*m3_s.*cos(TH3_s).*(1.0./2.0)+L1Y_s.*L2Y_s.*m2_s.*cos(TH1_s.*2.0+TH2_s).*(1.0./2.0)+L1Y_s.*L2Y_s.*m3_s.*cos(TH1_s.*2.0+TH2_s)+L1Y_s.*L3Y_s.*m3_s.*cos(TH1_s.*2.0+TH2_s+TH3_s).*(1.0./2.0)+L1Y_s.*L3Y_s.*m3_s.*cos(TH2_s+TH3_s).*(1.0./2.0)+L2Y_s.*L3Y_s.*m3_s.*cos(TH1_s.*2.0+TH2_s.*2.0+TH3_s).*(1.0./2.0)],[4,4]);
if nargout > 1
    C = reshape([-L1Y_s.*L3Y_s.*TH2_s_D.*m3_s.*sin(TH2_s+TH3_s)-L1Y_s.*L3Y_s.*TH3_s_D.*m3_s.*sin(TH2_s+TH3_s)-L1Y_s.*L2Y_s.*TH2_s_D.*m2_s.*sin(TH2_s)-L1Y_s.*L2Y_s.*TH2_s_D.*m3_s.*sin(TH2_s).*2.0-L2Y_s.*L3Y_s.*TH3_s_D.*m3_s.*sin(TH3_s),L1Y_s.*L3Y_s.*TH1_s_D.*m3_s.*sin(TH2_s+TH3_s).*(1.0./2.0)+L1Y_s.*L2Y_s.*TH1_s_D.*m2_s.*sin(TH2_s).*(1.0./2.0)+L1Y_s.*L2Y_s.*TH1_s_D.*m3_s.*sin(TH2_s)-L2Y_s.*L3Y_s.*TH3_s_D.*m3_s.*sin(TH3_s),L3Y_s.*m3_s.*(L1Y_s.*TH1_s_D.*sin(TH2_s+TH3_s)+L2Y_s.*TH1_s_D.*sin(TH3_s)+L2Y_s.*TH2_s_D.*sin(TH3_s).*2.0).*(1.0./2.0),TH4_s_D.*(L3Y_s.^2.*m3_s.*sin(TH1_s.*2.0+TH2_s.*2.0+TH3_s.*2.0).*4.0-L3Z_s.^2.*m3_s.*sin(TH1_s.*2.0+TH2_s.*2.0+TH3_s.*2.0)+L1Y_s.^2.*m1_s.*sin(TH1_s.*2.0).*4.0+L1Y_s.^2.*m2_s.*sin(TH1_s.*2.0).*1.2e1+L1Y_s.^2.*m3_s.*sin(TH1_s.*2.0).*1.2e1-L1Z_s.^2.*m1_s.*sin(TH1_s.*2.0)+L2Y_s.^2.*m2_s.*sin(TH1_s.*2.0+TH2_s.*2.0).*4.0+L2Y_s.^2.*m3_s.*sin(TH1_s.*2.0+TH2_s.*2.0).*1.2e1-L2Z_s.^2.*m2_s.*sin(TH1_s.*2.0+TH2_s.*2.0)+L1Y_s.*L2Y_s.*m2_s.*sin(TH1_s.*2.0+TH2_s).*1.2e1+L1Y_s.*L2Y_s.*m3_s.*sin(TH1_s.*2.0+TH2_s).*2.4e1+L1Y_s.*L3Y_s.*m3_s.*sin(TH1_s.*2.0+TH2_s+TH3_s).*1.2e1+L2Y_s.*L3Y_s.*m3_s.*sin(TH1_s.*2.0+TH2_s.*2.0+TH3_s).*1.2e1).*(-1.0./1.2e1),L1Y_s.*L3Y_s.*TH2_s_D.*m3_s.*sin(TH2_s+TH3_s).*(-1.0./2.0)-L1Y_s.*L3Y_s.*TH3_s_D.*m3_s.*sin(TH2_s+TH3_s)-L1Y_s.*L2Y_s.*TH2_s_D.*m2_s.*sin(TH2_s).*(1.0./2.0)-L1Y_s.*L2Y_s.*TH2_s_D.*m3_s.*sin(TH2_s)-L2Y_s.*L3Y_s.*TH3_s_D.*m3_s.*sin(TH3_s),-L2Y_s.*L3Y_s.*TH3_s_D.*m3_s.*sin(TH3_s),L2Y_s.*L3Y_s.*TH2_s_D.*m3_s.*sin(TH3_s).*(1.0./2.0),TH4_s_D.*(L3Y_s.^2.*m3_s.*sin(TH1_s.*2.0+TH2_s.*2.0+TH3_s.*2.0).*4.0-L3Z_s.^2.*m3_s.*sin(TH1_s.*2.0+TH2_s.*2.0+TH3_s.*2.0)+L2Y_s.^2.*m2_s.*sin(TH1_s.*2.0+TH2_s.*2.0).*4.0+L2Y_s.^2.*m3_s.*sin(TH1_s.*2.0+TH2_s.*2.0).*1.2e1-L2Z_s.^2.*m2_s.*sin(TH1_s.*2.0+TH2_s.*2.0)+L1Y_s.*L2Y_s.*m2_s.*sin(TH2_s).*6.0+L1Y_s.*L2Y_s.*m3_s.*sin(TH2_s).*1.2e1+L1Y_s.*L2Y_s.*m2_s.*sin(TH1_s.*2.0+TH2_s).*6.0+L1Y_s.*L2Y_s.*m3_s.*sin(TH1_s.*2.0+TH2_s).*1.2e1+L1Y_s.*L3Y_s.*m3_s.*sin(TH1_s.*2.0+TH2_s+TH3_s).*6.0+L1Y_s.*L3Y_s.*m3_s.*sin(TH2_s+TH3_s).*6.0+L2Y_s.*L3Y_s.*m3_s.*sin(TH1_s.*2.0+TH2_s.*2.0+TH3_s).*1.2e1).*(-1.0./1.2e1),L3Y_s.*TH3_s_D.*m3_s.*(L1Y_s.*sin(TH2_s+TH3_s)+L2Y_s.*sin(TH3_s)).*(-1.0./2.0),L2Y_s.*L3Y_s.*TH3_s_D.*m3_s.*sin(TH3_s).*(-1.0./2.0),0.0,TH4_s_D.*m3_s.*(L3Y_s.^2.*sin(TH1_s.*2.0+TH2_s.*2.0+TH3_s.*2.0).*4.0-L3Z_s.^2.*sin(TH1_s.*2.0+TH2_s.*2.0+TH3_s.*2.0)+L1Y_s.*L3Y_s.*sin(TH1_s.*2.0+TH2_s+TH3_s).*6.0+L1Y_s.*L3Y_s.*sin(TH2_s+TH3_s).*6.0+L2Y_s.*L3Y_s.*sin(TH1_s.*2.0+TH2_s.*2.0+TH3_s).*6.0+L2Y_s.*L3Y_s.*sin(TH3_s).*6.0).*(-1.0./1.2e1),TH4_s_D.*(L3Y_s.^2.*m3_s.*sin(TH1_s.*2.0+TH2_s.*2.0+TH3_s.*2.0).*4.0-L3Z_s.^2.*m3_s.*sin(TH1_s.*2.0+TH2_s.*2.0+TH3_s.*2.0)+L1Y_s.^2.*m1_s.*sin(TH1_s.*2.0).*4.0+L1Y_s.^2.*m2_s.*sin(TH1_s.*2.0).*1.2e1+L1Y_s.^2.*m3_s.*sin(TH1_s.*2.0).*1.2e1-L1Z_s.^2.*m1_s.*sin(TH1_s.*2.0)+L2Y_s.^2.*m2_s.*sin(TH1_s.*2.0+TH2_s.*2.0).*4.0+L2Y_s.^2.*m3_s.*sin(TH1_s.*2.0+TH2_s.*2.0).*1.2e1-L2Z_s.^2.*m2_s.*sin(TH1_s.*2.0+TH2_s.*2.0)+L1Y_s.*L2Y_s.*m2_s.*sin(TH1_s.*2.0+TH2_s).*1.2e1+L1Y_s.*L2Y_s.*m3_s.*sin(TH1_s.*2.0+TH2_s).*2.4e1+L1Y_s.*L3Y_s.*m3_s.*sin(TH1_s.*2.0+TH2_s+TH3_s).*1.2e1+L2Y_s.*L3Y_s.*m3_s.*sin(TH1_s.*2.0+TH2_s.*2.0+TH3_s).*1.2e1).*(1.0./2.4e1),TH4_s_D.*(L3Y_s.^2.*m3_s.*sin(TH1_s.*2.0+TH2_s.*2.0+TH3_s.*2.0).*4.0-L3Z_s.^2.*m3_s.*sin(TH1_s.*2.0+TH2_s.*2.0+TH3_s.*2.0)+L2Y_s.^2.*m2_s.*sin(TH1_s.*2.0+TH2_s.*2.0).*4.0+L2Y_s.^2.*m3_s.*sin(TH1_s.*2.0+TH2_s.*2.0).*1.2e1-L2Z_s.^2.*m2_s.*sin(TH1_s.*2.0+TH2_s.*2.0)+L1Y_s.*L2Y_s.*m2_s.*sin(TH2_s).*6.0+L1Y_s.*L2Y_s.*m3_s.*sin(TH2_s).*1.2e1+L1Y_s.*L2Y_s.*m2_s.*sin(TH1_s.*2.0+TH2_s).*6.0+L1Y_s.*L2Y_s.*m3_s.*sin(TH1_s.*2.0+TH2_s).*1.2e1+L1Y_s.*L3Y_s.*m3_s.*sin(TH1_s.*2.0+TH2_s+TH3_s).*6.0+L1Y_s.*L3Y_s.*m3_s.*sin(TH2_s+TH3_s).*6.0+L2Y_s.*L3Y_s.*m3_s.*sin(TH1_s.*2.0+TH2_s.*2.0+TH3_s).*1.2e1).*(1.0./2.4e1),TH4_s_D.*m3_s.*(L3Y_s.^2.*sin(TH1_s.*2.0+TH2_s.*2.0+TH3_s.*2.0).*4.0-L3Z_s.^2.*sin(TH1_s.*2.0+TH2_s.*2.0+TH3_s.*2.0)+L1Y_s.*L3Y_s.*sin(TH1_s.*2.0+TH2_s+TH3_s).*6.0+L1Y_s.*L3Y_s.*sin(TH2_s+TH3_s).*6.0+L2Y_s.*L3Y_s.*sin(TH1_s.*2.0+TH2_s.*2.0+TH3_s).*6.0+L2Y_s.*L3Y_s.*sin(TH3_s).*6.0).*(1.0./2.4e1),0.0],[4,4]);
end
if nargout > 2
    K = reshape([0.0,0.0,0.0,0.0,0.0,0.0,0.0,0.0,0.0,0.0,0.0,0.0,0.0,0.0,0.0,0.0],[4,4]);
end
if nargout > 3
    G = [g_s.*(L2Y_s.*m2_s.*cos(TH1_s+TH2_s)+L2Y_s.*m3_s.*cos(TH1_s+TH2_s).*2.0+L1Y_s.*m1_s.*cos(TH1_s)+L1Y_s.*m2_s.*cos(TH1_s).*2.0+L1Y_s.*m3_s.*cos(TH1_s).*2.0+L3Y_s.*m3_s.*cos(TH1_s+TH2_s+TH3_s)).*(1.0./2.0);L3Y_s.*g_s.*m3_s.*cos(TH1_s+TH2_s+TH3_s).*(1.0./2.0)+L2Y_s.*g_s.*m2_s.*cos(TH1_s+TH2_s).*(1.0./2.0)+L2Y_s.*g_s.*m3_s.*cos(TH1_s+TH2_s);L3Y_s.*g_s.*m3_s.*cos(TH1_s+TH2_s+TH3_s).*(1.0./2.0);0.0];
end
if nargout > 4
    Q = [taum1_s-TH1_s_D.*b1_s;taum2_s-TH2_s_D.*b2_s;taum3_s-TH3_s_D.*b3_s;taum4_s-TH4_s_D.*b4_s];
end

== matlab function bh_CONTROL_4dof_manip_swing_balance/MODE CONTROLLER/STATE_CONTROL/DO_BALANCE_calcs/DO_BALANCE_sys/MATLAB Function ==
  data: u input; y output
function y = fcn(u)
coder.extrinsic('wrapToPi');
y = 0;
y = wrapToPi(u);

== matlab function bh_CONTROL_4dof_manip_swing_balance/SIMULINK_MODEL/inside_MCKGQ/Subsystem1/MATLAB Function ==
  data: M input; the_cond output
function the_cond = COND(M)
%#codegen

the_cond = cond(M);

end

== matlab function bh_CONTROL_4dof_manip_swing_balance/MODE CONTROLLER/LINK2_YZ_TO_CMD_BUS/GET_ready_calcs/CALC_THETA_DOT ==
  data: J input; TH_DOT output; XY_DOT input; lambda_sq input; alt_TH_DOT output
function [TH_DOT, alt_TH_DOT] = calc_TH_DOT(J, XY_DOT, lambda_sq)
%#codegen

TH_DOT     = zeros(2,1);
alt_TH_DOT = zeros(2,1);

    %% so our problem is this:
    %     J*q_dot = x_dot
    %
    % so a solution is:
    %
    %      q_dot = pinv(J) * x_dot
    
    TH_DOT = pinv(J) * XY_DOT;

    %% we can also penalise the q_dot by applying a weight to it.
    %  this will give us a solution where we get a "smaller" q_dot.  This
    %  acts as a "dampening" agent ... and we notice it most at startup.
    
    % consider solving the REGULARISED problem
    %     [       J_mxn  ] * q_dot =  [ x_dot ]
    %     [lamb^2*I_nxn  ]            [ 0_nx1 ]
    %
    % which we'll wite as:
    %
    %              new_A * q_dot = new_b
    %
    % so a solution is:
    %
    %      q_dot = pinv(new_A) * new_b
    
    [m, n]     = size(J); 
    I_mat      = eye( n ); 
    new_A      = [ J;
                   lambda_sq * I_mat];

    new_b      = [ XY_DOT;
                   zeros(n,1) ];
    %alt_TH_DOT = zeros(m,1);
    alt_TH_DOT = pinv( new_A  ) * new_b;
end

== matlab function bh_CONTROL_4dof_manip_swing_balance/MODE CONTROLLER/LINK2_YZ_TO_CMD_BUS/GET_ready_calcs/MATLAB Function ==
  data: J input; the_cond output
function the_cond = COND(J)
%#codegen

the_cond = cond(J);

end

== matlab function bh_CONTROL_4dof_manip_swing_balance/MODE CONTROLLER/LINK2_YZ_TO_CMD_BUS/GET_ready_calcs/THE_J ==
  data: L_1 input; the_J output; L_2 input; theta_1 input; theta_2 input
function the_J = THE_J(L_1,L_2,theta_1,theta_2)
%#codegen

%    This function was generated by the Symbolic Math Toolbox version 7.0.
%    05-Sep-2016 11:04:30

the_J = reshape([-L_2.*sin(theta_1+theta_2)-L_1.*sin(theta_1),L_2.*cos(theta_1+theta_2)+L_1.*cos(theta_1),-L_2.*sin(theta_1+theta_2),L_2.*cos(theta_1+theta_2)],[2,2]);

== matlab function bh_CONTROL_4dof_manip_swing_balance/MODE CONTROLLER/LINK2_YZ_TO_CMD_BUS/GET_ready_calcs/THE_XE_YE ==
  data: L_1 input; XE output; L_2 input; theta_1 input; theta_2 input; YE output
function [XE,YE] = THE_XEYE(L_1,L_2,theta_1,theta_2)
%#codegen

%    This function was generated by the Symbolic Math Toolbox version 7.0.
%    05-Sep-2016 11:23:53

XE = L_2.*cos(theta_1+theta_2)+L_1.*cos(theta_1);
if nargout > 1
    YE = L_2.*sin(theta_1+theta_2)+L_1.*sin(theta_1);
end

== stateflow chart bh_CONTROL_4dof_manip_swing_balance/MODE CONTROLLER/STATE_CONTROL/Chart ==
  state DO_POSE_READY
    exit: OUT_y_at_sw_start = INP_EFF_LINK2_y;
  state DO_SWING_UP
    exit:
    OUT_y_at_bal_start = INP_EFF_LINK2_y;
    OUT_yD_at_bal_start = INP_EFF_LINK2_y_D;
  state BIRTH
  state DO_BALANCE
  (default) -> BIRTH
  BIRTH -> DO_POSE_READY : [MLF_is_LINK_3_hanging_down]
  DO_POSE_READY -> DO_SWING_UP : [MLF_is_EFF_at_y_ready]
  DO_SWING_UP -> DO_BALANCE : [MLF_is_LINK_3_standing_upright]
  data: tf_val function_output; tf_val function_output; tf_val function_output; INP_EFF_LINK2_y input double size=1; INP_EFF_LINK2_y_D input double size=1; INP_LINK3_theta3 input double size=1; INP_LINK3_theta3_D input double size=1; INP_EFF_LINK2_y_GOAL input double size=1; BIRTH output boolean; DO_POSE_READY output boolean; DO_SWING_UP output boolean; DO_BALANCE output boolean; OUT_y_at_sw_start output size=1; OUT_y_at_bal_start output size=1; OUT_yD_at_bal_start output size=1
  function tf_val = MLF_is_LINK_3_hanging_down:
    | function tf_val = MLF_is_LINK_3_hanging_down
    | 
    | TH_diff     = (-pi/2) - INP_LINK3_theta3;
    | TH_DIFF_deg = TH_diff * 180/pi; 
    | 
    | TH_DOT_diff    = (0) - INP_LINK3_theta3_D;
    | TH_DOT_DOF_deg = TH_DOT_diff * 180/pi;
    | 
    | if( abs(TH_DIFF_deg) <= 1 && abs(TH_DOT_DOF_deg) < 1 )
    |     tf_val = true;
    | else
    |     tf_val = false;
    | end
  function tf_val = MLF_is_LINK_3_standing_upright:
    | function tf_val = MLF_is_LINK_3_standing_upright
    | 
    | tf_val = false;
    | 
    | TH_diff     = (pi/2) - INP_LINK3_theta3;
    | TH_DIFF_deg = TH_diff * 180/pi; 
    | 
    | if( abs(TH_DIFF_deg) <= 10  )
    |     tf_val = true;
    | end
    | 
    | % now check for -270 degrees
    | 
    | TH_diff     = (-3*pi/2) - INP_LINK3_theta3;
    | TH_DIFF_deg = TH_diff * 180/pi; 
    | 
    | if( abs(TH_DIFF_deg) <= 10  )
    |     tf_val = true;
    | end
  function tf_val = MLF_is_EFF_at_y_ready:
    | function tf_val = MLF_is_EFF_at_y_ready
    | 
    | y_diff = INP_EFF_LINK2_y_GOAL - INP_EFF_LINK2_y;
    | 
    | if( abs(y_diff) < 0.001 )
    |     tf_val = true;
    | else
    |     tf_val = false;
    | end

== matlab function bh_CONTROL_4dof_manip_swing_balance/MODE CONTROLLER/STATE_CONTROL/Subsystem/LINK2_EFF_YZ_from_THETA/THE_XE_YE ==
  data: L_1 input; XE output; L_2 input; theta_1 input; theta_2 input; YE output
function [XE,YE] = THE_XEYE(L_1,L_2,theta_1,theta_2)
%#codegen

%    This function was generated by the Symbolic Math Toolbox version 7.0.
%    05-Sep-2016 11:23:53

XE = L_2.*cos(theta_1+theta_2)+L_1.*cos(theta_1);
if nargout > 1
    YE = L_2.*sin(theta_1+theta_2)+L_1.*sin(theta_1);
end

== matlab function bh_CONTROL_4dof_manip_swing_balance/Create_PLANT_BUS/CALC_BUS/THE_A_EFF_and_O_and_G ==
  data: L1Y_s input; AF_pos_eff output; L2Y_s input; L3Y_s input; theta1 input; theta2 input; theta3 input; AF_pos_O1 output; AF_pos_O2 output; AF_pos_O3 output; AF_pos_G1 output; AF_pos_G2 output; AF_pos_G3 output
function [AF_pos_eff,AF_pos_O1,AF_pos_O2,AF_pos_O3,AF_pos_G1,AF_pos_G2,AF_pos_G3] = THE_A_EFF_and_O_and_G(L1Y_s,L2Y_s,L3Y_s,theta1,theta2,theta3)
%#codegen

%    This function was generated by the Symbolic Math Toolbox version 7.0.
%    15-Sep-2016 15:54:05

AF_pos_eff = [0.0;L2Y_s.*cos(theta1+theta2)+L1Y_s.*cos(theta1)+L3Y_s.*cos(theta1+theta2+theta3);L2Y_s.*sin(theta1+theta2)+L1Y_s.*sin(theta1)+L3Y_s.*sin(theta1+theta2+theta3)];
if nargout > 1
    AF_pos_O1 = [0.0;0.0;0.0];
end
if nargout > 2
    AF_pos_O2 = [0.0;L1Y_s.*cos(theta1);L1Y_s.*sin(theta1)];
end
if nargout > 3
    AF_pos_O3 = [0.0;L2Y_s.*cos(theta1+theta2)+L1Y_s.*cos(theta1);L2Y_s.*sin(theta1+theta2)+L1Y_s.*sin(theta1)];
end
if nargout > 4
    AF_pos_G1 = [0.0;L1Y_s.*cos(theta1).*(1.0./2.0);L1Y_s.*sin(theta1).*(1.0./2.0)];
end
if nargout > 5
    AF_pos_G2 = [0.0;L2Y_s.*cos(theta1+theta2).*(1.0./2.0)+L1Y_s.*cos(theta1);L2Y_s.*sin(theta1+theta2).*(1.0./2.0)+L1Y_s.*sin(theta1)];
end
if nargout > 6
    AF_pos_G3 = [0.0;L2Y_s.*cos(theta1+theta2)+L1Y_s.*cos(theta1)+L3Y_s.*cos(theta1+theta2+theta3).*(1.0./2.0);L2Y_s.*sin(theta1+theta2)+L1Y_s.*sin(theta1)+L3Y_s.*sin(theta1+theta2+theta3).*(1.0./2.0)];
end

== matlab function bh_CONTROL_4dof_manip_swing_balance/Create_PLANT_BUS/CALC_BUS/THE_W_EFF_and_O_and_G ==
  data: L1Y_s input; WF_pos_eff output; L2Y_s input; L3Y_s input; theta1 input; theta2 input; theta3 input; theta4 input; WF_pos_O1 output; WF_pos_O2 output; WF_pos_O3 output; WF_pos_G1 output; WF_pos_G2 output; WF_pos_G3 output
function [WF_pos_eff,WF_pos_O1,WF_pos_O2,WF_pos_O3,WF_pos_G1,WF_pos_G2,WF_pos_G3] = THE_W_EFF_and_O_and_G(L1Y_s,L2Y_s,L3Y_s,theta1,theta2,theta3,theta4)
%#codegen

%    This function was generated by the Symbolic Math Toolbox version 7.0.
%    15-Sep-2016 15:32:27

WF_pos_eff = [-sin(theta4).*(L2Y_s.*cos(theta1+theta2)+L1Y_s.*cos(theta1)+L3Y_s.*cos(theta1+theta2+theta3));cos(theta4).*(L2Y_s.*cos(theta1+theta2)+L1Y_s.*cos(theta1)+L3Y_s.*cos(theta1+theta2+theta3));L2Y_s.*sin(theta1+theta2)+L1Y_s.*sin(theta1)+L3Y_s.*sin(theta1+theta2+theta3)];
if nargout > 1
    WF_pos_O1 = [0.0;0.0;0.0];
end
if nargout > 2
    WF_pos_O2 = [-L1Y_s.*cos(theta1).*sin(theta4);L1Y_s.*cos(theta1).*cos(theta4);L1Y_s.*sin(theta1)];
end
if nargout > 3
    WF_pos_O3 = [-sin(theta4).*(L2Y_s.*cos(theta1+theta2)+L1Y_s.*cos(theta1));cos(theta4).*(L2Y_s.*cos(theta1+theta2)+L1Y_s.*cos(theta1));L2Y_s.*sin(theta1+theta2)+L1Y_s.*sin(theta1)];
end
if nargout > 4
    WF_pos_G1 = [L1Y_s.*cos(theta1).*sin(theta4).*(-1.0./2.0);L1Y_s.*cos(theta1).*cos(theta4).*(1.0./2.0);L1Y_s.*sin(theta1).*(1.0./2.0)];
end
if nargout > 5
    WF_pos_G2 = [-sin(theta4).*(L2Y_s.*cos(theta1+theta2).*(1.0./2.0)+L1Y_s.*cos(theta1));cos(theta4).*(L2Y_s.*cos(theta1+theta2).*(1.0./2.0)+L1Y_s.*cos(theta1));L2Y_s.*sin(theta1+theta2).*(1.0./2.0)+L1Y_s.*sin(theta1)];
end
if nargout > 6
    WF_pos_G3 = [-sin(theta4).*(L2Y_s.*cos(theta1+theta2)+L1Y_s.*cos(theta1)+L3Y_s.*cos(theta1+theta2+theta3).*(1.0./2.0));cos(theta4).*(L2Y_s.*cos(theta1+theta2)+L1Y_s.*cos(theta1)+L3Y_s.*cos(theta1+theta2+theta3).*(1.0./2.0));L2Y_s.*sin(theta1+theta2)+L1Y_s.*sin(theta1)+L3Y_s.*sin(theta1+theta2+theta3).*(1.0./2.0)];
end

== matlab function bh_CONTROL_4dof_manip_swing_balance/Create_PLANT_BUS/Subsystem1/MATLAB Function ==
  data: r input size=[3 1]; TQ output; F input size=[3 1]
function TQ = CROSS(r,F)
%#codegen

TQ = cross(r,F);

== matlab function bh_CONTROL_4dof_manip_swing_balance/Create_PLANT_BUS/Subsystem1/MATLAB Function1 ==
  data: r input size=[3 1]; TQ output; F input size=[3 1]
function TQ = CROSS(r,F)
%#codegen

TQ = cross(r,F);

== matlab function bh_CONTROL_4dof_manip_swing_balance/Create_PLANT_BUS/Subsystem1/MATLAB Function2 ==
  data: r input size=[3 1]; TQ output; F input size=[3 1]
function TQ = CROSS(r,F)
%#codegen

TQ = cross(r,F);

== matlab function bh_CONTROL_4dof_manip_swing_balance/Create_PLANT_BUS/Subsystem1/MATLAB Function3 ==
  data: r input size=[3 1]; TQ output; F input size=[3 1]
function TQ = CROSS(r,F)
%#codegen

TQ = cross(r,F);

== matlab function bh_CONTROL_4dof_manip_swing_balance/Create_PLANT_BUS/Subsystem1/MATLAB Function4 ==
  data: r input size=[3 1]; TQ output; F input size=[3 1]
function TQ = CROSS(r,F)
%#codegen

TQ = cross(r,F);

== matlab function bh_CONTROL_4dof_manip_swing_balance/Create_PLANT_BUS/Subsystem1/MATLAB Function5 ==
  data: r input size=[3 1]; TQ output; F input size=[3 1]
function TQ = CROSS(r,F)
%#codegen

TQ = cross(r,F);

== matlab function bh_CONTROL_4dof_manip_swing_balance/MODE CONTROLLER/STATE_CONTROL/DO_SWING_UP_calcs/MATLAB Function ==
  data: t input; TH input; the_yo output; TH_DOT input; mass3 input; L3y input; b3_damp input; Io3_xx input; a0 input; k input; E_goal output; E output
function [the_yo, E_goal, E]  = fcn(t, TH, TH_DOT, mass3, L3y, b3_damp, Io3_xx, a0, k)

persistent last_yo 
persistent tf_is_doing_phase_1
persistent last_theta_dot
persistent t_at_end_phase_1
persistent t_start

if( isempty(last_yo) )
    last_yo             = 0;
    tf_is_doing_phase_1 = true;
    last_theta_dot      = 0;
    t_at_end_phase_1    = 0;
    t_start             = t;
end

my_t          = t - t_start;
the_yo        = 0;
    theta     = TH;   
    theta_dot = TH_DOT;

BETA          = theta + pi/2;
wn            = sqrt(mass3*9.81*L3y/Io3_xx); 
T             = 1/(wn/(2*pi));

h             =   0.5 * L3y * sin(theta);  
E_goal        = mass3 * 9.81 *  (L3y/2);

PE            = mass3 * 9.81 * h;
KE            = 0.5 * Io3_xx * (theta_dot^2);
E             = PE;   %E     = PE + KE;
E_diff        = E - E_goal;

phi           = atan2( -1*theta_dot/wn, BETA);

if(my_t<=3*T)
    the_yo         = a0 * sin(  1.0*my_t*wn );
    last_yo        = the_yo;
    last_theta_dot = theta_dot;
    return
end


if(tf_is_doing_phase_1==true)

    if(sign(theta_dot) ~= sign(last_theta_dot) )
        tf_is_doing_phase_1 = false;
        t_at_end_phase_1    = my_t;
    end
        
    return
end

%k         = 2.17; %2.2; %2;
Y1        = a0 * sin(  1.0*my_t*wn );
Y2        = a0 * sin(k*phi -pi ) ;
the_yo    = Y2;

== matlab function bh_CONTROL_4dof_manip_swing_balance/SL_VIEW/XYZ_EFF_COMPARE /THE_XE_YE ==
  data: L_1 input; XE output; L_2 input; theta_1 input; theta_2 input; YE output
function [XE,YE] = THE_XEYE(L_1,L_2,theta_1,theta_2)
%#codegen

%    This function was generated by the Symbolic Math Toolbox version 7.0.
%    05-Sep-2016 11:23:53

XE = L_2.*cos(theta_1+theta_2)+L_1.*cos(theta_1);
if nargout > 1
    YE = L_2.*sin(theta_1+theta_2)+L_1.*sin(theta_1);
end
